simulink model "GalvoTransferFuncFeedbackDelay"  (R2013a)
settings: Solver=ode45  StartTime=0.0  StopTime=init.StopTime  FixedStep=1e-6  MinStep=init.MinStepSize  RelTol=1e-3
undefined symbols (not defined in the file or in its folder): init, MinStepSize, PID, TsSens, TsSens2
libraries: simulink x2
settings Model: BufferReuse=off  Creator=mainster  LastModifiedBy=mainster
settings SolverCC: InitialStep=init.MinStepSize
settings DataIOCC: SignalLoggingSaveFormat=ModelDataLogs
settings OptimizationCC: OptimizeBlockIOStorage=off  BufferReuse=off  ExpressionFolding=off  ExpressionDepthLimit=2147483647  LocalBlockOutputs=off
settings DebuggingCC: FcnCallInpInsideContextMsg=UseLocalSettings
settings GRTTargetCC: CombineOutputUpdateFcns=off  GRTInterface=on

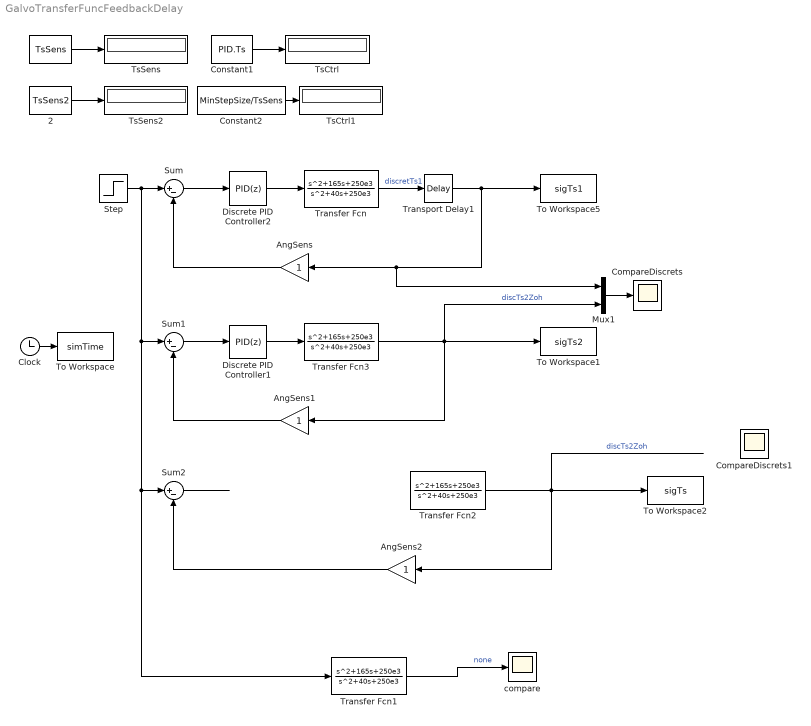
== system GalvoTransferFuncFeedbackDelay ==
  " " : Constant  Value=TsSens
  2 : Constant  Value=TsSens2
  AngSens : Gain  SampleTime=init.TsSens
  AngSens1 : Gain  SampleTime=init.TsSens2
  AngSens2 : Gain  SampleTime=init.TsSens2
  Clock : Clock
  CompareDiscrets : Scope
      settings: ShowLegends=on  TimeRange=0.05  YMin=0.9  YMax=1.1
  CompareDiscrets1 : Scope
      settings: ShowLegends=on  TimeRange=0.05  YMin=0.9  YMax=1.1
  Constant1 : Constant  Value=PID.Ts
  Constant2 : Constant  Value=MinStepSize/TsSens
  Discrete PID Controller1 : simulink/Continuous/PID Controller  Controller=PID  TimeDomain=Discrete-time  SampleTime=PID.Ts  IntegratorMethod=Forward Euler  FilterMethod=Forward Euler  Form=Parallel  P=PID.P  I=PID.I  D=PID.D  N=PID.N  InitialConditionSource=internal  InitialConditionForIntegrator=0  InitialConditionForFilter=0  ExternalReset=none  LimitOutput=off  UpperSaturationLimit=inf  LowerSaturationLimit=-inf  LinearizeAsGain=off  AntiWindupMode=none  Kb=1  TrackingMode=off  Kt=1  PParamMin=[]  PParamMax=[]  IParamMin=[]  IParamMax=[]  DParamMin=[]  DParamMax=[]  NParamMin=[]  NParamMax=[]  KbParamMin=[]  KbParamMax=[]  KtParamMin=[]  KtParamMax=[]  POutMin=[]  POutMax=[]  IOutMin=[]  IOutMax=[]  DOutMin=[]  DOutMax=[]  NOutMin=[]  NOutMax=[]  KbOutMin=[]  KbOutMax=[]  KtOutMin=[]  KtOutMax=[]  IntegratorOutMin=[]  IntegratorOutMax=[]  FilterOutMin=[]  FilterOutMax=[]  SumOutMin=[]  SumOutMax=[]  SumI1OutMin=[]  SumI1OutMax=[]  SumI2OutMin=[]  SumI2OutMax=[]  SumI3OutMin=[]  SumI3OutMax=[]  SumDOutMin=[]  SumDOutMax=[]  SaturationOutMin=[]  SaturationOutMax=[]  IntegratorContinuousStateAttributes=''  IntegratorStateMustResolveToSignalObject=off  IntegratorRTWStateStorageClass=Auto  FilterContinuousStateAttributes=''  FilterStateMustResolveToSignalObject=off  FilterRTWStateStorageClass=Auto
  Discrete PID Controller2 : simulink/Continuous/PID Controller  Controller=PID  TimeDomain=Discrete-time  SampleTime=PID.Ts  IntegratorMethod=Forward Euler  FilterMethod=Forward Euler  Form=Parallel  P=PID.P  I=PID.I  D=PID.D  N=PID.N  InitialConditionSource=internal  InitialConditionForIntegrator=0  InitialConditionForFilter=0  ExternalReset=none  LimitOutput=off  UpperSaturationLimit=inf  LowerSaturationLimit=-inf  LinearizeAsGain=off  AntiWindupMode=none  Kb=1  TrackingMode=off  Kt=1  PParamMin=[]  PParamMax=[]  IParamMin=[]  IParamMax=[]  DParamMin=[]  DParamMax=[]  NParamMin=[]  NParamMax=[]  KbParamMin=[]  KbParamMax=[]  KtParamMin=[]  KtParamMax=[]  POutMin=[]  POutMax=[]  IOutMin=[]  IOutMax=[]  DOutMin=[]  DOutMax=[]  NOutMin=[]  NOutMax=[]  KbOutMin=[]  KbOutMax=[]  KtOutMin=[]  KtOutMax=[]  IntegratorOutMin=[]  IntegratorOutMax=[]  FilterOutMin=[]  FilterOutMax=[]  SumOutMin=[]  SumOutMax=[]  SumI1OutMin=[]  SumI1OutMax=[]  SumI2OutMin=[]  SumI2OutMax=[]  SumI3OutMin=[]  SumI3OutMax=[]  SumDOutMin=[]  SumDOutMax=[]  SaturationOutMin=[]  SaturationOutMax=[]  IntegratorContinuousStateAttributes=''  IntegratorStateMustResolveToSignalObject=off  IntegratorRTWStateStorageClass=Auto  FilterContinuousStateAttributes=''  FilterStateMustResolveToSignalObject=off  FilterRTWStateStorageClass=Auto
  Mux1 : Mux  Inputs=2
  Step : Step  Time=0.01  SampleTime=0
  Sum : Sum  Inputs=|+-  SampleTime=init.TsSens
  Sum1 : Sum  Inputs=|+-  SampleTime=init.TsSens2
  Sum2 : Sum  Inputs=|+-  SampleTime=init.TsSens2
  To Workspace : ToWorkspace  VariableName=simTime  SampleTime=-1  SaveFormat=Timeseries
  To Workspace1 : ToWorkspace  VariableName=sigTs2  SampleTime=-1  SaveFormat=Structure
  To Workspace2 : ToWorkspace  VariableName=sigTs  SampleTime=-1  SaveFormat=Structure
  To Workspace5 : ToWorkspace  VariableName=sigTs1  SampleTime=-1  SaveFormat=Structure
  Transfer Fcn{,1..3} (4 alike) : TransferFcn  Numerator=[1 165 250e3]  Denominator=[1 40 250e3]
  Transport Delay1 : TransportDelay  DelayTime=init.DelayTime
  TsCtrl : Display
      settings: Format=short_e
  TsCtrl1 : Display
      settings: Format=short_e
  TsSens : Display
      settings: Format=short_e
  TsSens2 : Display
      settings: Format=short_e
  compare : Scope
      settings: TickLabels=on  ShowLegends=on  TimeRange=0.05  YMin=0  YMax=1.4  SaveName=ScopeData2
  wires:
  Sum/1 -> Discrete PID Controller2/1
  Transfer Fcn/1 -> Transport Delay1/1  "discretTs1"
  Discrete PID Controller2/1 -> Transfer Fcn/1
  AngSens/1 -> Sum/2
  Constant1/1 -> TsCtrl/1
  " "/1 -> TsSens/1
  Sum1/1 -> Discrete PID Controller1/1
  Discrete PID Controller1/1 -> Transfer Fcn3/1
  AngSens1/1 -> Sum1/2
  Mux1/1 -> CompareDiscrets/1
  2/1 -> TsSens2/1
  Constant2/1 -> TsCtrl1/1
  Clock/1 -> To Workspace/1
  Transport Delay1/1 -> Mux1/1, AngSens/1, To Workspace5/1
  Transfer Fcn3/1 -> AngSens1/1, Mux1/2, To Workspace1/1  "discTs2Zoh"
  Transfer Fcn1/1 -> compare/1  "none"
  Step/1 -> Sum/1, Sum1/1, Sum2/1, Transfer Fcn1/1
  Sum2/1 -> ?
  ? -> Transfer Fcn2/1
  AngSens2/1 -> Sum2/2
  Transfer Fcn2/1 -> AngSens2/1, To Workspace2/1  "discTs2Zoh"
